simulink subsystem "get_adj_obstacles_Subsystem"  (R2024a)
settings: Solver=VariableStepAuto  StartTime=0.0  StopTime=10.0  RelTol=1e-3
settings Model: Creator=User  LastModifiedBy=User

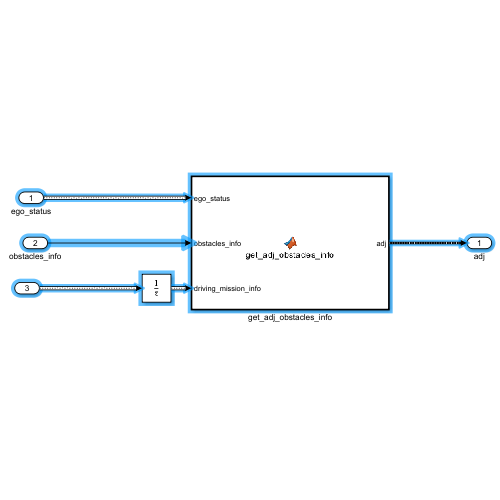
[thumbnail: Simulink's stored preview of the top-level diagram]
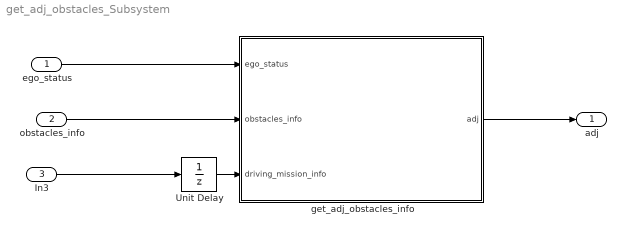
== system get_adj_obstacles_Subsystem ==
  ego_status : Inport
  obstacles_info : Inport  Port=2
  In3 : Inport  Port=3
  Unit Delay : UnitDelay  SampleTime=-1  HasFrameUpgradeWarning=on
  get_adj_obstacles_info : MATLAB Function  TreatAsAtomicUnit=on
  adj : Outport
  wires:
  Unit Delay/1 -> get_adj_obstacles_info/3(driving_mission_info)
  In3/1 -> Unit Delay/1
  ego_status/1 -> get_adj_obstacles_info/1(ego_status)
  get_adj_obstacles_info/1(adj) -> adj/1
  obstacles_info/1 -> get_adj_obstacles_info/2(obstacles_info)

== matlab function get_adj_obstacles_Subsystem/get_adj_obstacles_info ==
  settings: sampleTime=0.05
  data: ego_status input; obstacles_info input [3..10]; adj output size=[8 10]; driving_mission_info input
function adj = get_adj_obstacles_info(ego_status, obstacles_info, driving_mission_info)
    % obstacles_info   : Nx matrix or struct (each obstacle row = one vehicle)
    %                    columns assumed: [X, Y, Vx, Vy, Ax, Ay, Yaw, Yawrate]

    % disp('--------')
    % disp(obstacles_info);
    % disp('--------')
    % disp('Vehicle_position')
    % disp(vehicle_position);
    % disp('--------')

    mission_state = driving_mission_info.missionState;
    if mission_state >= 3
        adj = zeros(3, 10);
        return;
    end
    
    dist_threshhold = 30.0;
    
    ego_x = ego_status.ego_X;
    ego_y = ego_status.ego_Y;

    X = obstacles_info(:,1);
    Y = obstacles_info(:,2);

    % 거리 계산
    dx = X - ego_x;
    dy = Y - ego_y;
    dist = dx.^2 + dy.^2;

    % threshold 안에 있는 인덱스
    idx = dist < dist_threshhold^2;

    % 필터링된 장애물 정보
    adj = obstacles_info(idx, :);
    
    % disp(idx);
    % if ~isempty(adj)
    %     disp('-----')
    %     disp(adj(1, :));
    % end
end
